simulink model "task6"  (R2017a)
settings: Solver=VariableStepAuto  StartTime=0.0  StopTime=25  RelTol=1e-3
values from neighbouring files (symbols this model uses):
  A = [-8.8487+(a-b)/5 -0.0399 -5.55+(c+d)/10 3.5846 ... (first row only)    [initialize.m]
  B = [0.0564+b/(10+c) 0.0319 ... (first row only)    [initialize.m]
  C = [-3.2988 -2.1932+(10*c+d)/(100+5*a) 0.037 -0.0109 ... (first row only)    [initialize.m]
  K1 = K_LQR(:,1:4)    [MIMO_servo_control_with_observer.m]    (also in MIMO_servo_control_without_observer.m; last_task.m)
  K2 = K_LQR(:,5:6)    [MIMO_servo_control_with_observer.m]    (also in MIMO_servo_control_without_observer.m; last_task.m)
  Y_SP = C*X_SP    [last_task.m]
settings Model: Creator=lenovo  LastModifiedBy=lenovo

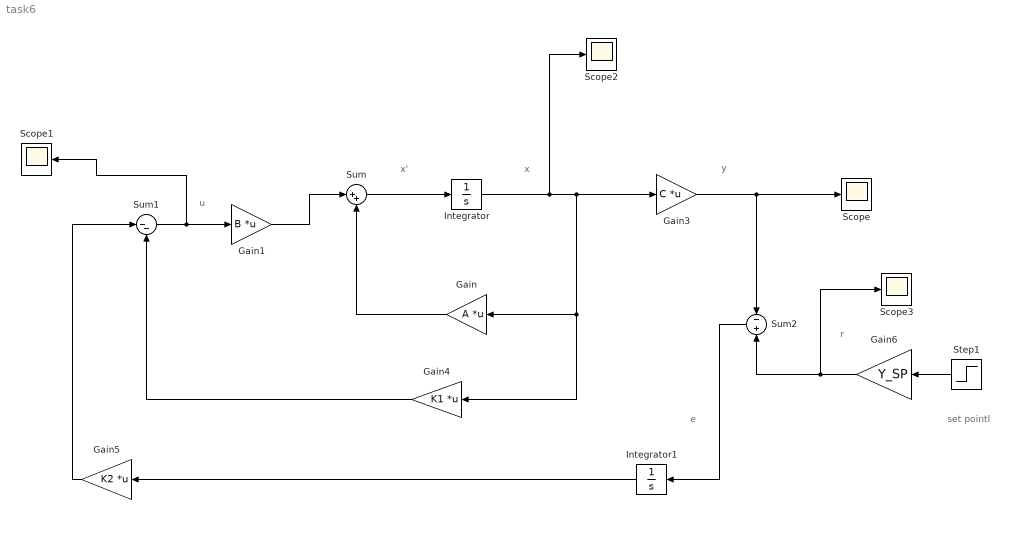
== system task6 ==
  note: e
  note: set pointl
  note: y
  note: r
  note: x
  note: x'
  note: u
  Gain : Gain  Gain=A  Multiplication=Matrix(K*u)
  Gain1 : Gain  Gain=B  Multiplication=Matrix(K*u)
  Gain3 : Gain  Gain=C  Multiplication=Matrix(K*u)
  Gain4 : Gain  Gain=K1  Multiplication=Matrix(K*u)
  Gain5 : Gain  Gain=K2  Multiplication=Matrix(K*u)
  Gain6 : Gain  Gain=Y_SP
  Integrator : Integrator  InitialCondition=[0.5;-0.1;0.3;-0.8]
  Integrator1 : Integrator
  Scope{,1..3} (4 alike) : Scope
  Step1 : Step  Time=0  Before=[0;0]  After=[1;1]  SampleTime=0  VectorParams1D=off
  Sum : Sum  Inputs=|++
  Sum1 : Sum  Inputs=|--
  Sum2 : Sum  Inputs=-|+
  wires:
  Sum2/1 -> Integrator1/1
  Gain4/1 -> Sum1/2
  Sum/1 -> Integrator/1
  Gain3/1 -> Scope/1, Sum2/1
  Integrator1/1 -> Gain5/1
  Integrator/1 -> Scope2/1, Gain3/1, Gain4/1, Gain/1
  Gain5/1 -> Sum1/1
  Sum1/1 -> Scope1/1, Gain1/1
  Step1/1 -> Gain6/1
  Gain6/1 -> Scope3/1, Sum2/2
  Gain/1 -> Sum/2
  Gain1/1 -> Sum/1
